simulink model "mcb_pmsm_foc_abs_current_loop"  (R2024a)
settings: Solver=FixedStepAuto  StartTime=0.0  StopTime=2  FixedStep=1e-6  RelTol=1e-3
undefined symbols (not defined in the file or in its folder): current, motor
libraries: mcbcontrolslib x7, simulink_extras x3, slpidlib x2, spsDCVoltageSourceLib x1, eePwmGeneratorTwoLevel x1, spsUniversalBridgeLib x1, spsPermanentMagnetSynchronousMachineLib x1, spsThreePhaseVIMeasurementLib x1, spspowerguiLib x1
settings Model: Creator=dark  LastModifiedBy=dark

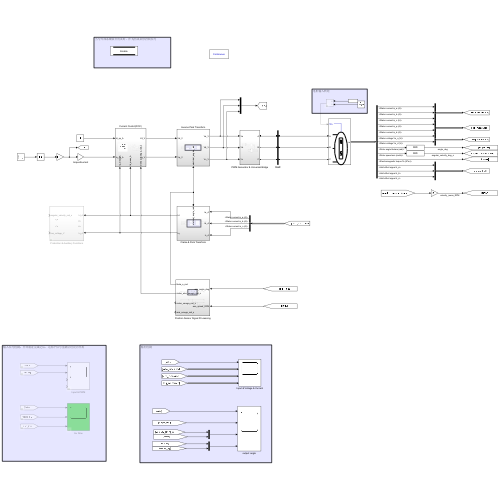
[thumbnail: Simulink's stored preview of the top-level diagram]
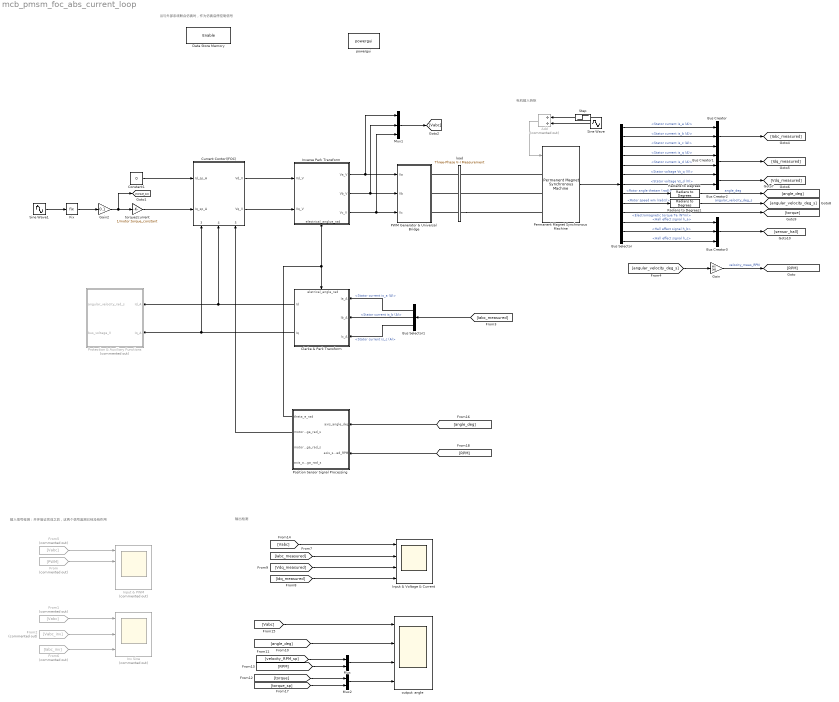
== system mcb_pmsm_foc_abs_current_loop ==
  note: 电机输入转矩
  note: 当与外部系统联合仿真时，作为仿真启停控制信号
  note: 输出检测
  note: 输入信号检测：开环验证完成之后，这两个信号监测已经没有作用
  Add : Sum  Commented=on
  Bus Creator : BusCreator  Inputs=3
  Bus Creator1 : BusCreator  Inputs=2
  Bus Creator2 : BusCreator  Inputs=2
  Bus Creator3 : BusCreator  Inputs=3
  Bus Selector : BusSelector  OutputSignals=Stator current is_a (A),Stator current is_b (A),Stator current is_c (A),Stator current is_q (A),Stator current is_d (A),Stator voltage Vs_q (V),Stator voltage Vs_d (V),Rotor angle thetam (rad),Rotor speed wm (rad/s),Electromagnetic torque Te (N*m),Hall effect signal h_a,Hall effect signal h_b,Hall effect signal h_c
  Bus Selector1 : BusSelector  OutputSignals=Stator current is_a (A),Stator current is_b (A),Stator current is_c (A)
  Clarke & Park Transform : Subsystem
      settings: PortSchema="{\"entries\":[{\"content\":{\"sides\":[{\"content\":{\"connectorIds\":[\"Out1\",\"Out2\"]},\"type\":\"ConnectorPlacement.EquallySpacedRectSide\",\"uuid\":\"8f5ea7de-e3a5-4729-b10e-8648bf1336c0\"},{\"content\":{\"connectorIds\":[\"In2\",\"In3\",\"In4\"],\"side\":\"RIGHT\"},\"type\":\"ConnectorPlacement.EquallySpacedRectSide\",\"uuid\":\"bbc5fc22-58ea-4d3d-90f4-5c6a0078be5c\"},{\"content\":{\"connectorIds\":[\"In1\"],\"side\":\"TOP\"},\"type\":\"ConnectorPlacement.EquallySpacedRectSide\",\"uuid\":\"61ad1e16-6f66-442a-8711-29b4040ed318\"}]},\"type\":\"ConnectorPlacement.EquallySpacedConnector\",\"uuid\":\"7625cfb7-138f-4210-9cc7-b054236901ec\"}],\"packageUris\":[\"http://schema.mathworks.com/mf0/Connector/R2020b\"],\"version\":\"1.0\"}"
  Constant1 : Constant  Value=0
  Current Contorl(FOC) : Subsystem
      settings: PortSchema="{\"entries\":[{\"content\":{\"sides\":[{\"content\":{\"connectorIds\":[\"In1\",\"In2\"]},\"type\":\"ConnectorPlacement.EquallySpacedRectSide\",\"uuid\":\"8f5ea7de-e3a5-4729-b10e-8648bf1336c0\"},{\"content\":{\"connectorIds\":[\"Out1\",\"Out2\"],\"side\":\"RIGHT\"},\"type\":\"ConnectorPlacement.EquallySpacedRectSide\",\"uuid\":\"bbc5fc22-58ea-4d3d-90f4-5c6a0078be5c\"},{\"content\":{\"side\":\"TOP\"},\"type\":\"ConnectorPlacement.EquallySpacedRectSide\",\"uuid\":\"61ad1e16-6f66-442a-8711-29b4040ed318\"},{\"content\":{\"connectorIds\":[\"In3\",\"In4\",\"In5\"],\"side\":\"BOTTOM\"},\"type\":\"ConnectorPlacement.EquallySpacedRectSide\",\"uuid\":\"11568d81-d3e5-4cf0-a61c-40e52990d6e7\"}]},\"type\":\"ConnectorPlacement.EquallySpacedConnector\",\"uuid\":\"7625cfb7-138f-4210-9cc7-b054236901ec\"}],\"packageUris\":[\"http://schema.mathworks.com/mf0/Connector/R2020b\"],\"version\":\"1.0\"}"
  Data Store Memory : DataStoreMemory  DataStoreName=Enable  WriteAfterWriteMsg=warning  InitialValue=1  ShowAdditionalParam=off  OutDataTypeStr=boolean
  Fix : Rounding  Operator=fix
  From : From  Commented=on  GotoTag=PWM
  From1 : From  Commented=on  GotoTag=Vabc
  From2 : From  Commented=on  GotoTag=Vabc_inv  TagVisibility=global
  From5 : From  Commented=on  GotoTag=Vabc
  From6 : From  Commented=on  GotoTag=Iabc_inv  TagVisibility=global
  Gain : Gain  Gain=60 / 360
  Gain2 : Gain  Gain=0.1
  Input & PWM : Scope  Commented=on  NumInputPorts=4
  Input & Voltage & Current : Scope  NumInputPorts=4
  Inv Sine : Scope  Commented=on  NumInputPorts=3
  Inverse Park Transform : Subsystem
      settings: PortSchema="{\"entries\":[{\"content\":{\"sides\":[{\"content\":{\"connectorIds\":[\"In1\",\"In2\"]},\"type\":\"ConnectorPlacement.EquallySpacedRectSide\",\"uuid\":\"a02395ac-75c0-4856-959c-e255f60cf021\"},{\"content\":{\"connectorIds\":[\"Out1\",\"Out2\",\"Out3\"],\"side\":\"RIGHT\"},\"type\":\"ConnectorPlacement.EquallySpacedRectSide\",\"uuid\":\"9eafc65f-7434-4d14-b216-6fa625ac6e03\"},{\"content\":{\"side\":\"TOP\"},\"type\":\"ConnectorPlacement.EquallySpacedRectSide\",\"uuid\":\"619f9ca2-00b2-4830-addc-46008419189b\"},{\"content\":{\"connectorIds\":[\"In3\"],\"side\":\"BOTTOM\"},\"type\":\"ConnectorPlacement.EquallySpacedRectSide\",\"uuid\":\"9a5dc0ea-6fa9-4e2d-93f5-5e384ac5faa7\"}]},\"type\":\"ConnectorPlacement.EquallySpacedConnector\",\"uuid\":\"2cf4530c-aae1-4e2c-824f-90ca12c00a06\"}],\"packageUris\":[\"http://schema.mathworks.com/mf0/Connector/R2020b\"],\"version\":\"1.0\"}"
  Mux : Mux  Inputs=2
  Mux1 : Mux  Inputs=3
  Mux2 : Mux  Inputs=2
  PWM Generator & Universal Bridge : Subsystem
  Permanent Magnet Synchronous Machine : spsPermanentMagnetSynchronousMachineLib/Permanent Magnet Synchronous Machine  NbPhases=3  FluxDistribution=Sinusoidal  RotorType=Salient-pole  MechanicalLoad=Torque Tm  PresetModel=No  ShowDetailedParameters=on  MeasurementBus=off  Resistance=motor.phase_resistance  Inductance=8.5e-3  dqInductances=[motor.phase_inductance, motor.phase_inductance]  La=0.000395  MachineConstant=Torque Constant (N.m / A_peak)  Flux=0.0078901  VoltageCst=7.1555  TorqueCst=motor.torque_constant  Flat=120  Mechanical=[motor.inertia motor.friction_damping_factor motor.pole_pairs 0]  PolePairs=4  InitialConditions=[0,0, 0,0]  InitialConditions5ph=[0 0 0 0 0 0]  RefAngle=Aligned with phase A axis (original Park)  IterativeDiscreteModel=Trapezoidal non iterative  TsBlock=-1  TsPowergui=0
  Position Sensor Signal Processing : Subsystem
      settings: PortSchema="{\"entries\":[{\"content\":{\"sides\":[{\"content\":{\"connectorIds\":[\"Out1\",\"Out2\",\"Out3\",\"Out4\"]},\"type\":\"ConnectorPlacement.EquallySpacedRectSide\",\"uuid\":\"fa7647be-1c66-4470-a30c-b3ca7d023db7\"},{\"content\":{\"connectorIds\":[\"In1\",\"In2\"],\"side\":\"RIGHT\"},\"type\":\"ConnectorPlacement.EquallySpacedRectSide\",\"uuid\":\"1ad87a77-5065-44e2-877c-562c1ba61661\"},{\"content\":{\"side\":\"TOP\"},\"type\":\"ConnectorPlacement.EquallySpacedRectSide\",\"uuid\":\"cb7afcba-6dc8-40ee-b8e6-8d1e642ae95d\"}]},\"type\":\"ConnectorPlacement.EquallySpacedConnector\",\"uuid\":\"59faac42-ead8-4d3d-a16a-460d437d8ea5\"}],\"packageUris\":[\"http://schema.mathworks.com/mf0/Connector/R2020b\"],\"version\":\"1.0\"}"
  Protection & Auxiliary Functions : Subsystem  Commented=on
      settings: PortSchema="{\"entries\":[{\"content\":{\"sides\":[{\"content\":{\"connectorIds\":[\"In1\",\"In2\"]},\"type\":\"ConnectorPlacement.EquallySpacedRectSide\",\"uuid\":\"7b4d6b93-1ce9-4e0c-abad-a47a6899df6c\"},{\"content\":{\"connectorIds\":[\"In3\",\"In4\"],\"side\":\"RIGHT\"},\"type\":\"ConnectorPlacement.EquallySpacedRectSide\",\"uuid\":\"d4cf6bf2-fc47-46ce-a267-e5931389b5f3\"},{\"content\":{\"side\":\"TOP\"},\"type\":\"ConnectorPlacement.EquallySpacedRectSide\",\"uuid\":\"5d917ce9-fbe2-4b0c-8b11-30f3f5ab2e3d\"}]},\"type\":\"ConnectorPlacement.EquallySpacedConnector\",\"uuid\":\"7aed4540-46f4-4bb4-951a-5ed091990878\"}],\"packageUris\":[\"http://schema.mathworks.com/mf0/Connector/R2020b\"],\"version\":\"1.0\"}"
  Radians to Degrees : simulink_extras/Transformations/Radians to Degrees
  Radians to Degrees1 : simulink_extras/Transformations/Radians to Degrees
  Sine Wave : Sin  Amplitude=0.1  Frequency=2*pi*10  SampleTime=0
  Sine Wave1 : Sin  Amplitude=2  Frequency=2*pi*10  SampleTime=0
  Step : Step  Time=0.2  After=0.05  SampleTime=0
  load : spsThreePhaseVIMeasurementLib/Three-Phase V-I Measurement  VoltageMeasurement=phase-to-phase  SetLabelV=on  LabelV=Vabc_inv  Vpu=off  VpuLL=off  CurrentMeasurement=yes  SetLabelI=on  LabelI=Iabc_inv  Ipu=off  Pbase=1e3  Vbase=380  OutputType=Magnitude  PhasorSimulation=off  PSBequivalent=0
  output: angle : Scope  NumInputPorts=4
  powergui : spspowerguiLib/powergui  Priority=1  SimulationMode=Continuous  SampleTime=50e-6  frequency=60  Iterations=50  frequencyindice=0  Pbase=100e6  ErrMax=1e-4  UnitsV=kV  UnitsW=MW  buscounter=0  FunctionMessages=off  echomessages=off  EnableUseOfTLC=off  CurrentSourceSwitches=off  DisableSnubberDevices=off  DisableRonSwitches=off  DisableVfSwitches=off  DisplayEquations=off  AutomaticDiscreteSolvers=off  SolverType=Tustin/Backward Euler (TBE)  Interpol=off  ExternalGateDelay=off  methode=off  Ts=100  x0status=blocks  SPID=on  SwTol=0  HookPort=off  NonlinearTolerance=1e-4  nMaxIteration=100  ContinueOnMaxIteration=off  RestoreLinks=warning  ResistiveCurrentMeasurement=off  Frange=[0:2:500]  Ylog=off  Xlog=on  ShowGrid=off  save=off  variable=ZData  structure=0  ZoomFFT=off  StartTime=0.0  cycles=1  DisplayStyle=1  fundamental=60  FreqAxis=off  MaxFrequency=1000  frequencyindicesteady=1  RmsSteady=1  display=off
  torque2current : Gain  Gain=1/motor.torque_constant
  wires:
  Permanent Magnet Synchronous Machine/1 -> Bus Selector/1
  Bus Selector/1 -> Bus Creator/1  "<Stator current is_a (A)>"
  Bus Selector/2 -> Bus Creator/2  "<Stator current is_b (A)>"
  Bus Selector/3 -> Bus Creator/3  "<Stator current is_c (A)>"
  From1/1 -> Inv Sine/1
  From6/1 -> Inv Sine/3
  From2/1 -> Inv Sine/2
  Bus Creator/1 -> [Iabc_measured]
  Bus Selector/4 -> Bus Creator1/1  "<Stator current is_q (A)>"
  Bus Selector/5 -> Bus Creator1/2  "<Stator current is_d (A)>"
  Bus Creator1/1 -> [Idq_measured]
  Bus Selector/10 -> [torque]  "<Electromagnetic torque Te (N*m)>"
  Bus Selector/8 -> Radians to Degrees/1  "<Rotor angle thetam (rad)>"
  Bus Selector/9 -> Radians to Degrees1/1  "<Rotor speed wm (rad/s)>"
  Bus Selector/6 -> Bus Creator2/1  "<Stator voltage Vs_q (V)>"
  Bus Selector/7 -> Bus Creator2/2  "<Stator voltage Vs_d (V)>"
  Bus Creator2/1 -> [Vdq_measured]
  Bus Creator3/1 -> [sensor_hall]
  Bus Selector/11 -> Bus Creator3/1  "<Hall effect signal h_a>"
  Bus Selector/12 -> Bus Creator3/2  "<Hall effect signal h_b>"
  Bus Selector/13 -> Bus Creator3/3  "<Hall effect signal h_c>"
  [Idq_measured] -> Input & Voltage & Current/4
  [Vdq_measured] -> Input & Voltage & Current/3
  [Iabc_measured] -> Input & Voltage & Current/2
  [Vabc] -> Input & Voltage & Current/1
  Radians to Degrees/1 -> [angle_deg]  "angle_deg"
  Radians to Degrees1/1 -> [angular_velocity_deg_s]  "angular_velocity_deg_s"
  [angle_deg] -> output: angle/2
  [Vabc] -> output: angle/1
  From5/1 -> Input & PWM/1
  From/1 -> Input & PWM/2
  Add/1 -> Permanent Magnet Synchronous Machine/1
  Step/1 -> Add/1
  Sine Wave/1 -> Add/2
  [angular_velocity_deg_s] -> Gain/1
  Gain/1 -> [RPM]  "velocity_meas_RPM"
  Mux/1 -> output: angle/3
  [velocity_RPM_sp] -> Mux/1
  [RPM] -> Mux/2
  [Iabc_measured] -> Bus Selector1/1
  Bus Selector1/2 -> Clarke & Park Transform/3(Ib_A)  "<Stator current is_b (A)>"
  Bus Selector1/1 -> Clarke & Park Transform/2(Ia_A)  "<Stator current is_a (A)>"
  Bus Selector1/3 -> Clarke & Park Transform/4(Ic_A)  "<Stator current is_c (A)>"
  Current Contorl(FOC)/2(Vq_V) -> Inverse Park Transform/2(Vq_V)
  Current Contorl(FOC)/1(Vd_V) -> Inverse Park Transform/1(Vd_V)
  Inverse Park Transform/3(Vc_V) -> Mux1/3, PWM Generator & Universal Bridge/3(Vc)
  Inverse Park Transform/2(Vb_V) -> Mux1/2, PWM Generator & Universal Bridge/2(Vb)
  Inverse Park Transform/1(Va_V) -> Mux1/1, PWM Generator & Universal Bridge/1(Va)
  Clarke & Park Transform/1(Id) -> Protection & Auxiliary Functions/3(Id_A), Current Contorl(FOC)/4(Id_meas_A)
  Clarke & Park Transform/2(Iq) -> Protection & Auxiliary Functions/4(Iq_A), Current Contorl(FOC)/3(Iq_meas_A)
  Position Sensor Signal Processing/1(theta_e_rad) -> Inverse Park Transform/3(electrical_anglue_rad), Clarke & Park Transform/1(eletrical_angle_rad)
  [RPM] -> Position Sensor Signal Processing/2(axis_speed_RPM)
  [angle_deg] -> Position Sensor Signal Processing/1(axis_angle_deg)
  Constant1/1 -> Current Contorl(FOC)/1(Id_sp_A)
  Mux1/1 -> [Vabc]
  Sine Wave1/1 -> Fix/1
  torque2current/1 -> Current Contorl(FOC)/2(Iq_sp_A)
  Position Sensor Signal Processing/2(motor_elec_omega_rad_s) -> Current Contorl(FOC)/5(eletrical_omega_rad_s)
  Fix/1 -> Gain2/1
  Gain2/1 -> [torque_sp], torque2current/1
  Mux2/1 -> output: angle/4
  [torque] -> Mux2/1
  [torque_sp] -> Mux2/2
  connections:
  load/RConn3 -- Permanent Magnet Synchronous Machine/LConn3
  Permanent Magnet Synchronous Machine/LConn1 -- load/RConn1
  Permanent Magnet Synchronous Machine/LConn2 -- load/RConn2
  load/LConn1 -- PWM Generator & Universal Bridge/RConn1
  load/LConn2 -- PWM Generator & Universal Bridge/RConn2
  load/LConn3 -- PWM Generator & Universal Bridge/RConn3

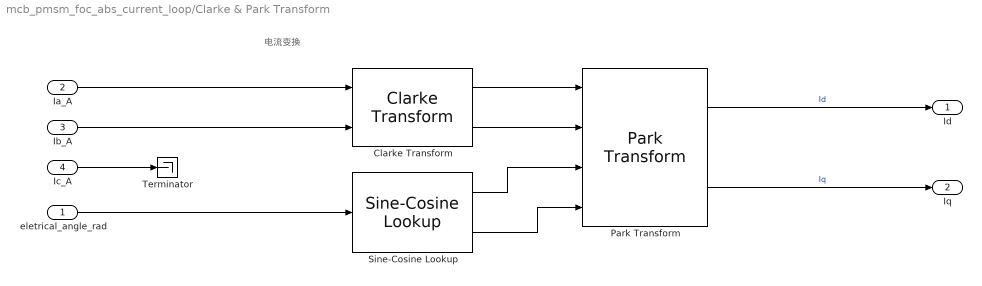
== system mcb_pmsm_foc_abs_current_loop/Clarke & Park Transform ==
  note: 电流变换
  eletrical_angle_rad : Inport
  Ia_A : Inport  Port=2
  Ib_A : Inport  Port=3
  Ic_A : Inport  Port=4
  Clarke Transform : mcbcontrolslib/Clarke Transform  VariantControl=Variant2  PhaseInput=Two inputs  EnPowerInv=off
      settings: LibrarySourceBlock=mcblib/Controls/Math Transforms/Clarke Transform
  Park Transform : mcbcontrolslib/Park Transform  PhaseInput=Two inputs  AxisAlignment=D-axis  ThetaInput=Sine and Cosine electrical position  AngleInput=Per-unit  N_points=1024
      settings: LibrarySourceBlock=mcblib/Controls/Math Transforms/Park Transform
  Sine-Cosine Lookup : mcbcontrolslib/Sine-Cosine Lookup  AngleInput=Radians  N_points=1024  DatatypeInput=Inherit from input  Datatype=single
      settings: LibrarySourceBlock=mcblib/Controls/Math Transforms/Sine-Cosine Lookup
  Terminator : Terminator
  Id : Outport
  Iq : Outport  Port=2
  wires:
  Clarke Transform/1 -> Park Transform/1
  eletrical_angle_rad/1 -> Sine-Cosine Lookup/1
  Clarke Transform/2 -> Park Transform/2
  Sine-Cosine Lookup/2 -> Park Transform/4
  Sine-Cosine Lookup/1 -> Park Transform/3
  Park Transform/1 -> Id/1  "Id"
  Park Transform/2 -> Iq/1  "Iq"
  Ic_A/1 -> Terminator/1
  Ib_A/1 -> Clarke Transform/2
  Ia_A/1 -> Clarke Transform/1

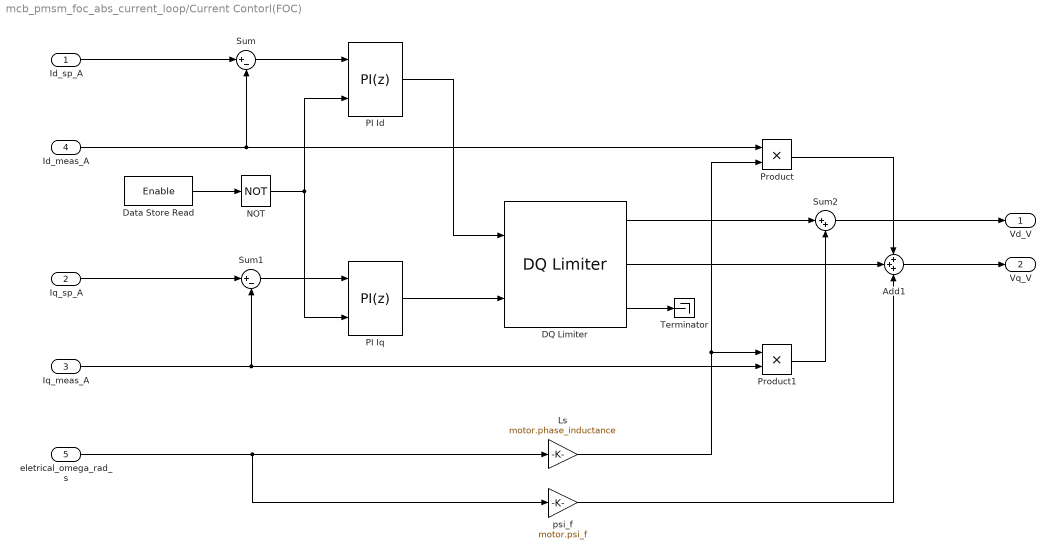
== system mcb_pmsm_foc_abs_current_loop/Current Contorl(FOC) ==
  Id_sp_A : Inport
  Iq_sp_A : Inport  Port=2
  Iq_meas_A : Inport  Port=3
  Id_meas_A : Inport  Port=4
  eletrical_omega_rad_s : Inport  Port=5
  Add1 : Sum  Inputs=+++
  DQ Limiter : mcbcontrolslib/DQ Limiter  satMethodInputType=Specify via dialog  satMethodSelected=D-Q equivalence  satLimitInputType=Specify via dialog  Vmax=24
      settings: LibrarySourceBlock=mcbhdllib/Controls/Control Reference/DQ Limiter
  Data Store Read : DataStoreRead  DataStoreName=Enable  IndexOptions=Index vector (dialog)  Indices=1  OutputSizes=1
  Ls : Gain  Gain=motor.phase_inductance
  NOT : Logic  Operator=NOT  IconShape=distinctive  AllPortsSameDT=off  OutDataTypeStr=boolean
  PI Id : slpidlib/PID Controller  Controller=PI  Form=Parallel  TimeDomain=Discrete-time  UseExternalTs=off  SampleTime=-1  IntegratorMethod=Forward Euler  FilterMethod=Forward Euler  ControllerParametersSource=internal  P=current.kp  I=current.ki  UseKiTs=off  D=0  UseExternalDerivativeSource=off  N=100  UseFilter=on  TunerSelectOption=Transfer Function Based (PID Tuner App)  InitialConditionSource=internal  InitialConditionForIntegrator=0  InitialConditionForFilter=0  DifferentiatorICPrevScaledInput=0  ExternalReset=level  TrackingMode=off  Kt=1  LimitOutput=off  SatLimitsSource=internal  UpperSaturationLimit=7.81  LowerSaturationLimit=-7.81  LinearizeAsGain=off  AntiWindupMode=clamping  Kb=1  LimitIntegrator=off  UpperIntegratorSaturationLimit=inf  LowerIntegratorSaturationLimit=-inf  POutMin=[]  POutMax=[]  IOutMin=[]  IOutMax=[]  DOutMin=[]  DOutMax=[]  NOutMin=[]  NOutMax=[]  SumOutMin=[]  SumOutMax=[]  SaturationOutMin=[]  SaturationOutMax=[]  PParamMin=[]  PParamMax=[]  IParamMin=[]  IParamMax=[]  DParamMin=[]  DParamMax=[]  NParamMin=[]  NParamMax=[]  KbParamMin=[]  KbParamMax=[]  KtParamMin=[]  KtParamMax=[]  KbOutMin=[]  KbOutMax=[]  KtOutMin=[]  KtOutMax=[]  IntegratorOutMin=[]  IntegratorOutMax=[]  FilterOutMin=[]  FilterOutMax=[]  SumI1OutMin=[]  SumI1OutMax=[]  SumI2OutMin=[]  SumI2OutMax=[]  SumI3OutMin=[]  SumI3OutMax=[]  SumI4OutMin=[]  SumI4OutMax=[]  SumDOutMin=[]  SumDOutMax=[]  DifferentiatorOutMin=[]  DifferentiatorOutMax=[]  FilterDiffOutCoefMin=[]  FilterDiffOutCoefMax=[]  ReciprocalOutMin=[]  ReciprocalOutMax=[]  SumDenOutMin=[]  SumDenOutMax=[]  SumNumOutMin=[]  SumNumOutMax=[]  DivideOutMin=[]  DivideOutMax=[]  UdiffTsProdOutMin=[]  UdiffTsProdOutMax=[]  NTsProdOutMin=[]  NTsProdOutMax=[]  UintegralTsProdOutMin=[]  UintegralTsProdOutMax=[]  UngainTsProdOutMin=[]  UngainTsProdOutMax=[]  ClampingZeroOutDataTypeStr=Inherit: Inherit via back propagation  ClampingZeroOutMin=[]  ClampingZeroOutMax=[]  FilterDenConstantOutDataTypeStr=Inherit: Inherit via back propagation  FilterDenConstantOutMin=[]  FilterDenConstantOutMax=[]  PCopyOutDataTypeStr=Inherit: Inherit via back propagation  PCopyOutMin=[]  PCopyOutMax=[]  NCopyOutDataTypeStr=Inherit: Inherit via back propagation  NCopyOutMin=[]  NCopyOutMax=[]  IntegratorContinuousStateAttributes=''  IntegratorStateMustResolveToSignalObject=off  IntegratorRTWStateStorageClass=Auto  FilterContinuousStateAttributes=''  FilterStateMustResolveToSignalObject=off  FilterRTWStateStorageClass=Auto  ParallelPVariant=InternalParameters  IdealPVariant=Disabled  IVariant=InternalParameters  DVariant=Disabled  IntegratorVariant=Discrete  SatVariant=Disabled  AWVariant=Passthrough  PCopyVariant=Disabled  TRVariant=Disabled  FdbkBlocksVariant=Forward  IdealPFdbkVariant=Disabled  SatFdbkVariant=Disabled  DerivativeFilterVariant=Disabled  NVariant=Disabled  NCopyVariant=Disabled_SignalSpec  FilterICVariant=Disabled  IntegratorICVariant=InternalICs  ExternalResetVariant=ExternalReset  TRSumVariant=Passthrough  SumFdbkVariant=Disabled  SumVariant=Sum_PI  TsampFilterVariant=InternalTs  TsampNgainVariant=Passthrough  TsampIntegralVariant=Disabled_SignalSpec  ExternalSaturationOutDataTypeStr=Inherit: Same as second input  DerivativeSourceVariant=Disabled
  PI Iq : slpidlib/PID Controller  Controller=PI  Form=Parallel  TimeDomain=Discrete-time  UseExternalTs=off  SampleTime=-1  IntegratorMethod=Forward Euler  FilterMethod=Forward Euler  ControllerParametersSource=internal  P=current.kp  I=current.ki  UseKiTs=off  D=0  UseExternalDerivativeSource=off  N=100  UseFilter=on  TunerSelectOption=Transfer Function Based (PID Tuner App)  InitialConditionSource=internal  InitialConditionForIntegrator=0  InitialConditionForFilter=0  DifferentiatorICPrevScaledInput=0  ExternalReset=level  TrackingMode=off  Kt=1  LimitOutput=off  SatLimitsSource=internal  UpperSaturationLimit=inf  LowerSaturationLimit=-inf  LinearizeAsGain=on  AntiWindupMode=none  Kb=1  LimitIntegrator=off  UpperIntegratorSaturationLimit=inf  LowerIntegratorSaturationLimit=-inf  POutMin=[]  POutMax=[]  IOutMin=[]  IOutMax=[]  DOutMin=[]  DOutMax=[]  NOutMin=[]  NOutMax=[]  SumOutMin=[]  SumOutMax=[]  SaturationOutMin=[]  SaturationOutMax=[]  PParamMin=[]  PParamMax=[]  IParamMin=[]  IParamMax=[]  DParamMin=[]  DParamMax=[]  NParamMin=[]  NParamMax=[]  KbParamMin=[]  KbParamMax=[]  KtParamMin=[]  KtParamMax=[]  KbOutMin=[]  KbOutMax=[]  KtOutMin=[]  KtOutMax=[]  IntegratorOutMin=[]  IntegratorOutMax=[]  FilterOutMin=[]  FilterOutMax=[]  SumI1OutMin=[]  SumI1OutMax=[]  SumI2OutMin=[]  SumI2OutMax=[]  SumI3OutMin=[]  SumI3OutMax=[]  SumI4OutMin=[]  SumI4OutMax=[]  SumDOutMin=[]  SumDOutMax=[]  DifferentiatorOutMin=[]  DifferentiatorOutMax=[]  FilterDiffOutCoefMin=[]  FilterDiffOutCoefMax=[]  ReciprocalOutMin=[]  ReciprocalOutMax=[]  SumDenOutMin=[]  SumDenOutMax=[]  SumNumOutMin=[]  SumNumOutMax=[]  DivideOutMin=[]  DivideOutMax=[]  UdiffTsProdOutMin=[]  UdiffTsProdOutMax=[]  NTsProdOutMin=[]  NTsProdOutMax=[]  UintegralTsProdOutMin=[]  UintegralTsProdOutMax=[]  UngainTsProdOutMin=[]  UngainTsProdOutMax=[]  ClampingZeroOutDataTypeStr=Inherit: Inherit via back propagation  ClampingZeroOutMin=[]  ClampingZeroOutMax=[]  FilterDenConstantOutDataTypeStr=Inherit: Inherit via back propagation  FilterDenConstantOutMin=[]  FilterDenConstantOutMax=[]  PCopyOutDataTypeStr=Inherit: Inherit via back propagation  PCopyOutMin=[]  PCopyOutMax=[]  NCopyOutDataTypeStr=Inherit: Inherit via back propagation  NCopyOutMin=[]  NCopyOutMax=[]  IntegratorContinuousStateAttributes=''  IntegratorStateMustResolveToSignalObject=off  IntegratorRTWStateStorageClass=Auto  FilterContinuousStateAttributes=''  FilterStateMustResolveToSignalObject=off  FilterRTWStateStorageClass=Auto  ParallelPVariant=InternalParameters  IdealPVariant=Disabled  IVariant=InternalParameters  DVariant=Disabled  IntegratorVariant=Discrete  SatVariant=Disabled  AWVariant=Passthrough  PCopyVariant=Disabled  TRVariant=Disabled  FdbkBlocksVariant=Forward  IdealPFdbkVariant=Disabled  SatFdbkVariant=Disabled  DerivativeFilterVariant=Disabled  NVariant=Disabled  NCopyVariant=Disabled_SignalSpec  FilterICVariant=Disabled  IntegratorICVariant=InternalICs  ExternalResetVariant=ExternalReset  TRSumVariant=Passthrough  SumFdbkVariant=Disabled  SumVariant=Sum_PI  TsampFilterVariant=InternalTs  TsampNgainVariant=Passthrough  TsampIntegralVariant=Disabled_SignalSpec  ExternalSaturationOutDataTypeStr=Inherit: Same as second input  DerivativeSourceVariant=Disabled
  Product : Product
  Product1 : Product
  Sum : Sum  Inputs=|+-
  Sum1 : Sum  Inputs=|+-
  Sum2 : Sum  Inputs=|++
  Terminator : Terminator
  psi_f : Gain  Gain=motor.psi_f
  Vd_V : Outport
  Vq_V : Outport  Port=2
  wires:
  DQ Limiter/3 -> Terminator/1
  Data Store Read/1 -> NOT/1
  Sum/1 -> PI Id/1
  Sum1/1 -> PI Iq/1
  Id_sp_A/1 -> Sum/1
  Id_meas_A/1 -> Product/1, Sum/2
  eletrical_omega_rad_s/1 -> Ls/1, psi_f/1
  Iq_meas_A/1 -> Product1/2, Sum1/2
  Iq_sp_A/1 -> Sum1/1
  Ls/1 -> Product/2, Product1/1
  NOT/1 -> PI Iq/2, PI Id/2
  PI Id/1 -> DQ Limiter/1
  PI Iq/1 -> DQ Limiter/2
  DQ Limiter/2 -> Add1/2
  Add1/1 -> Vq_V/1
  Product1/1 -> Sum2/2
  Product/1 -> Add1/1
  psi_f/1 -> Add1/3
  Sum2/1 -> Vd_V/1
  DQ Limiter/1 -> Sum2/1

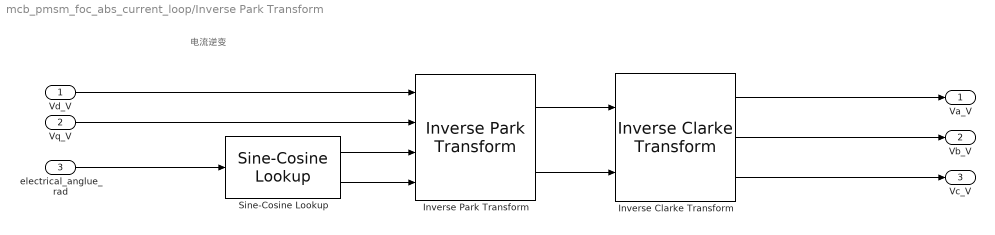
== system mcb_pmsm_foc_abs_current_loop/Inverse Park Transform ==
  note: 电流逆变
  Vd_V : Inport
  Vq_V : Inport  Port=2
  electrical_anglue_rad : Inport  Port=3
  Inverse Clarke Transform : mcbcontrolslib/Inverse Clarke Transform  PhaseInput=Two inputs  EnPowerInv=off
      settings: LibrarySourceBlock=mcblib/Controls/Math Transforms/Inverse Clarke Transform
  Inverse Park Transform : mcbcontrolslib/Inverse Park Transform  PhaseInput=Two inputs  AxisAlignment=D-axis  ThetaInput=Sine and Cosine electrical position  AngleInput=Radians  N_points=1024
      settings: LibrarySourceBlock=mcblib/Controls/Math Transforms/Inverse Park Transform
  Sine-Cosine Lookup : mcbcontrolslib/Sine-Cosine Lookup  AngleInput=Radians  N_points=1024  DatatypeInput=Inherit from input  Datatype=single
      settings: LibrarySourceBlock=mcblib/Controls/Math Transforms/Sine-Cosine Lookup
  Va_V : Outport
  Vb_V : Outport  Port=2
  Vc_V : Outport  Port=3
  wires:
  Inverse Park Transform/2 -> Inverse Clarke Transform/2
  Vd_V/1 -> Inverse Park Transform/1
  Inverse Park Transform/1 -> Inverse Clarke Transform/1
  Vq_V/1 -> Inverse Park Transform/2
  Sine-Cosine Lookup/1 -> Inverse Park Transform/3
  Sine-Cosine Lookup/2 -> Inverse Park Transform/4
  electrical_anglue_rad/1 -> Sine-Cosine Lookup/1
  Inverse Clarke Transform/1 -> Va_V/1
  Inverse Clarke Transform/2 -> Vb_V/1
  Inverse Clarke Transform/3 -> Vc_V/1

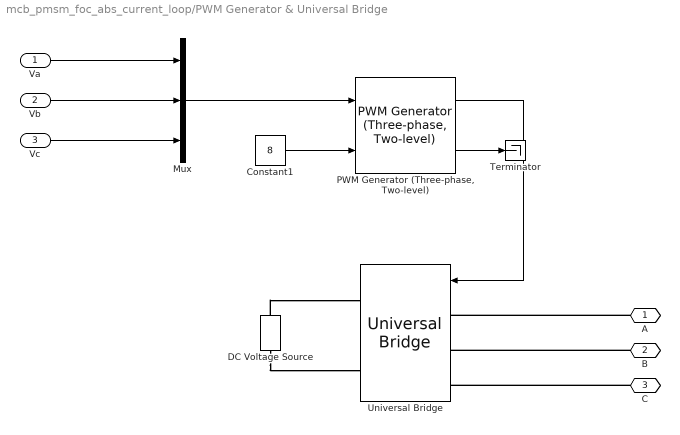
== system mcb_pmsm_foc_abs_current_loop/PWM Generator & Universal Bridge ==
  Va : Inport
  Vb : Inport  Port=2
  Vc : Inport  Port=3
  Constant1 : Constant  Value=8
  DC Voltage Source : spsDCVoltageSourceLib/DC Voltage Source  Amplitude=motor.voltage  Measurements=Voltage
  Mux : Mux  Inputs=3
  "PWM Generator (Three-phase, Two-level)" : eePwmGeneratorTwoLevel/PWM Generator (Three-phase, Two-level)  PWMMode=Continuous PWM (CPWM)  CPWMMode=SPWM: sinusoidal PWM  DPWMMode=60 DPWM: 60 degree discontinuous PWM  fsw=PWM.frequency  Ts=1e-6
      settings: LibrarySourceBlock=|
      | ee_sl_lib/Pulse Width
      | Modulation/PWM Generator
      | (Three-phase, Two-level)
  Terminator : Terminator
  Universal Bridge : spsUniversalBridgeLib/Universal Bridge  Arms=3  SnubberResistance=1e6  SnubberCapacitance=inf  Device=MOSFET / Diodes  Ron=1e-3  Lon=0  ForwardVoltages="[  0  0  ]"  ForwardVoltage=0  GTOparameters=[ 10e-6 , 20e-6 ]  IGBTparameters=[ 1e-6 , 2e-6 ]  Measurements=All voltages and currents  Measurements_2=None  converterType=Rectifier
  A : PMIOPort  Side=Right
  B : PMIOPort  Port=2  Side=Right
  C : PMIOPort  Port=3  Side=Right
  wires:
  "PWM Generator (Three-phase, Two-level)"/1 -> Universal Bridge/1
  Constant1/1 -> "PWM Generator (Three-phase, Two-level)"/2
  "PWM Generator (Three-phase, Two-level)"/2 -> Terminator/1
  Mux/1 -> "PWM Generator (Three-phase, Two-level)"/1
  Vc/1 -> Mux/3
  Vb/1 -> Mux/2
  Va/1 -> Mux/1
  connections:
  B/RConn1 -- Universal Bridge/LConn2
  DC Voltage Source/LConn1 -- Universal Bridge/RConn2
  DC Voltage Source/RConn1 -- Universal Bridge/RConn1
  C/RConn1 -- Universal Bridge/LConn3
  A/RConn1 -- Universal Bridge/LConn1

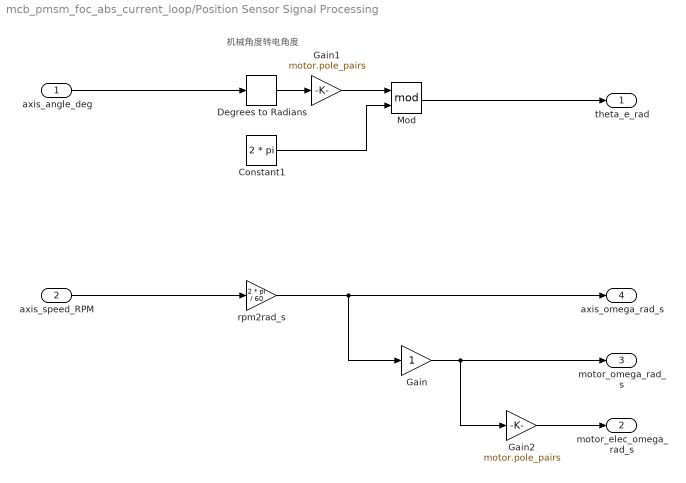
== system mcb_pmsm_foc_abs_current_loop/Position Sensor Signal Processing ==
  note: 机械角度转电角度
  axis_angle_deg : Inport
  axis_speed_RPM : Inport  Port=2
  Constant1 : Constant  Value=2 * pi
  Degrees to Radians : simulink_extras/Transformations/Degrees to Radians
  Gain : Gain
  Gain1 : Gain  Gain=motor.pole_pairs
  Gain2 : Gain  Gain=motor.pole_pairs
  Mod : Math  Operator=mod
  rpm2rad_s : Gain  Gain=2 * pi / 60
  theta_e_rad : Outport
  motor_elec_omega_rad_s : Outport  Port=2
  motor_omega_rad_s : Outport  Port=3
  axis_omega_rad_s : Outport  Port=4
  wires:
  axis_speed_RPM/1 -> rpm2rad_s/1
  Degrees to Radians/1 -> Gain1/1
  Gain1/1 -> Mod/1
  Constant1/1 -> Mod/2
  Mod/1 -> theta_e_rad/1
  axis_angle_deg/1 -> Degrees to Radians/1
  rpm2rad_s/1 -> Gain/1, axis_omega_rad_s/1
  Gain/1 -> Gain2/1, motor_omega_rad_s/1
  Gain2/1 -> motor_elec_omega_rad_s/1

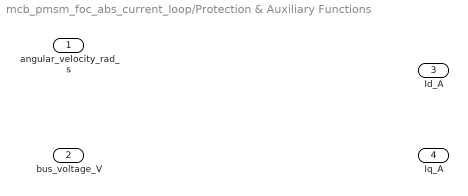
== system mcb_pmsm_foc_abs_current_loop/Protection & Auxiliary Functions ==
  angular_velocity_rad_s : Inport
  bus_voltage_V : Inport  Port=2
  Id_A : Inport  Port=3
  Iq_A : Inport  Port=4
